simulink library "INT_EngPrt_PrtLimOvht"  (R2016b)
settings: Solver=VariableStepAuto  StartTime=0.0  StopTime=10.0  RelTol=1e-3
settings Model: Creator=zhoutinglin  LastModifiedBy=zhoutinglin

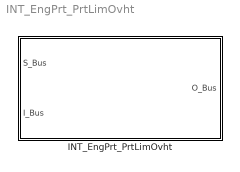
== system INT_EngPrt_PrtLimOvht ==
  INT_EngPrt_PrtLimOvht : Subsystem

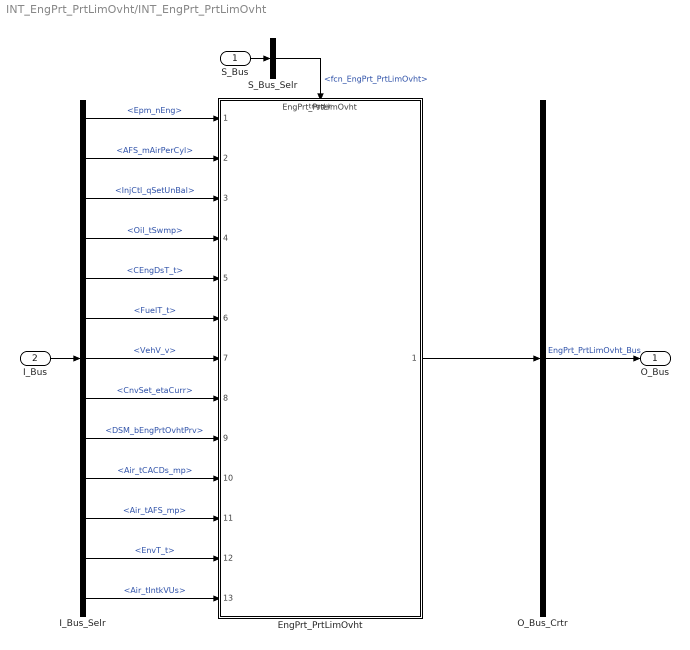
== system INT_EngPrt_PrtLimOvht/INT_EngPrt_PrtLimOvht ==
  S_Bus : Inport
  I_Bus : Inport  Port=2
  EngPrt_PrtLimOvht : ModelReference  ModelNameDialog=EngPrt_PrtLimOvht  SimulationMode=Normal  ModelReferenceVersion=1.26  TriggerPortName=function  TriggerPortTriggerType=function-call  TriggerPortStatesWhenEnabling=held
  I_Bus_Selr : BusSelector  OutputSignals=Epm_nEng,AFS_mAirPerCyl,InjCtl_qSetUnBal,Oil_tSwmp,CEngDsT_t,FuelT_t,VehV_v,CnvSet_etaCurr,DSM_bEngPrtOvhtPrv,Air_tCACDs_mp,Air_tAFS_mp,EnvT_t,Air_tIntkVUs
  O_Bus_Crtr : BusCreator  Inputs=1
  S_Bus_Selr : BusSelector  OutputSignals=fcn_EngPrt_PrtLimOvht
  O_Bus : Outport
  wires:
  S_Bus_Selr/1 -> EngPrt_PrtLimOvht/Trigger  "<fcn_EngPrt_PrtLimOvht>"
  S_Bus/1 -> S_Bus_Selr/1
  I_Bus/1 -> I_Bus_Selr/1
  I_Bus_Selr/1 -> EngPrt_PrtLimOvht/1  "<Epm_nEng>"
  I_Bus_Selr/2 -> EngPrt_PrtLimOvht/2  "<AFS_mAirPerCyl>"
  I_Bus_Selr/3 -> EngPrt_PrtLimOvht/3  "<InjCtl_qSetUnBal>"
  I_Bus_Selr/4 -> EngPrt_PrtLimOvht/4  "<Oil_tSwmp>"
  I_Bus_Selr/5 -> EngPrt_PrtLimOvht/5  "<CEngDsT_t>"
  I_Bus_Selr/6 -> EngPrt_PrtLimOvht/6  "<FuelT_t>"
  I_Bus_Selr/7 -> EngPrt_PrtLimOvht/7  "<VehV_v>"
  I_Bus_Selr/8 -> EngPrt_PrtLimOvht/8  "<CnvSet_etaCurr>"
  I_Bus_Selr/9 -> EngPrt_PrtLimOvht/9  "<DSM_bEngPrtOvhtPrv>"
  I_Bus_Selr/10 -> EngPrt_PrtLimOvht/10  "<Air_tCACDs_mp>"
  I_Bus_Selr/11 -> EngPrt_PrtLimOvht/11  "<Air_tAFS_mp>"
  I_Bus_Selr/12 -> EngPrt_PrtLimOvht/12  "<EnvT_t>"
  I_Bus_Selr/13 -> EngPrt_PrtLimOvht/13  "<Air_tIntkVUs>"
  O_Bus_Crtr/1 -> O_Bus/1  "EngPrt_PrtLimOvht_Bus"
  EngPrt_PrtLimOvht/1 -> O_Bus_Crtr/1
